simulink model "lista2_item_e_estimados"  (R2014b)
settings: Solver=ode45  StartTime=0.0  StopTime=Tsim  RelTol=1e-3
values from neighbouring files (symbols this model uses):
  T = 1    [sistema_lista2.m]
libraries: cstblocks x6
settings Model: Creator=Danilo  LastModifiedBy=Danilo

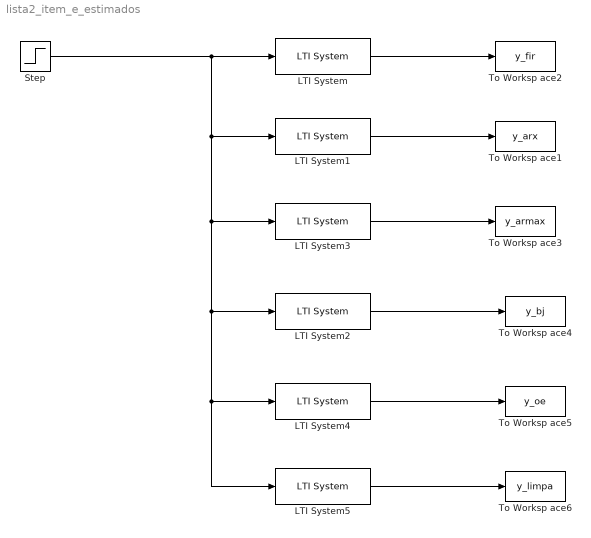
== system lista2_item_e_estimados ==
  LTI System : cstblocks/LTI System  sys=mdlfir  IC=[]
  LTI System1 : cstblocks/LTI System  sys=mdlarx  IC=[]
  LTI System2 : cstblocks/LTI System  sys=mdlbj  IC=[]
  LTI System3 : cstblocks/LTI System  sys=mdlarmax  IC=[]
  LTI System4 : cstblocks/LTI System  sys=mdloe  IC=[]
  LTI System5 : cstblocks/LTI System  sys=H  IC=[]
  Step : Step  Time=0  After=0.1  SampleTime=T
  To Worksp ace1 : ToWorkspace  VariableName=y_arx  SampleTime=T
  To Worksp ace2 : ToWorkspace  VariableName=y_fir  SampleTime=T
  To Worksp ace3 : ToWorkspace  VariableName=y_armax  SampleTime=T
  To Worksp ace4 : ToWorkspace  VariableName=y_bj  SampleTime=T
  To Worksp ace5 : ToWorkspace  VariableName=y_oe  SampleTime=T
  To Worksp ace6 : ToWorkspace  VariableName=y_limpa  SampleTime=T
  wires:
  Step/1 -> LTI System5/1, LTI System4/1, LTI System2/1, LTI System3/1, LTI System1/1, LTI System/1
  LTI System/1 -> To Worksp ace2/1
  LTI System1/1 -> To Worksp ace1/1
  LTI System3/1 -> To Worksp ace3/1
  LTI System2/1 -> To Worksp ace4/1
  LTI System4/1 -> To Worksp ace5/1
  LTI System5/1 -> To Worksp ace6/1
